simulink model "ADCS_model"  (R2019a)
settings: Solver=VariableStepAuto  StartTime=0.0  StopTime=10  RelTol=1e-3
undefined symbols (not defined in the file): A, As, c, Cd, f, G, J, JD_0, Jw, Ks, L, Ls, M, nut80, q
libraries: vrlib x5, dspmathops x1
(part 1 of 2)
settings Model: Creator=mario  LastModifiedBy=mario
settings DataIOCC: ReturnWorkspaceOutputs=off
settings DebuggingCC: ArithmeticOperatorsInVariantConditions=warning

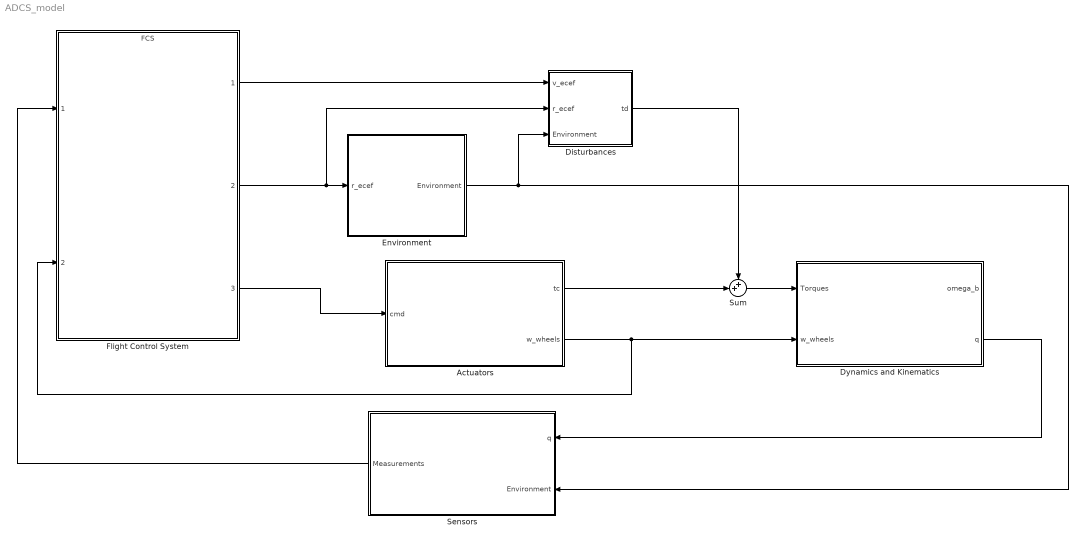
== system ADCS_model ==
  Actuators : Subsystem
  Disturbances : Subsystem
  "Dynamics and Kinematics " : Subsystem
  Environment : Subsystem
  Flight Control System : ModelReference  ModelNameDialog=FCS.slx  SimulationMode=Normal  ModelReferenceVersion=1.10
  Sensors : Subsystem
  Sum : Sum  Inputs=++|
  wires:
  "Dynamics and Kinematics "/2(q) -> Sensors/1(q)
  Sensors/1(Measurements) -> Flight Control System/1
  Disturbances/1(td) -> Sum/1
  Actuators/1(tc) -> Sum/2
  Environment/1(Environment) -> Sensors/2(Environment), Disturbances/3(Environment)
  Sum/1 -> "Dynamics and Kinematics "/1(Torques)
  Flight Control System/2 -> Environment/1(r_ecef), Disturbances/2("r_ecef ")
  Actuators/2(w_wheels) -> Flight Control System/2, "Dynamics and Kinematics "/2(w_wheels)
  Flight Control System/1 -> Disturbances/1(v_ecef)
  Flight Control System/3 -> Actuators/1(cmd)

== system ADCS_model/Actuators ==
  cmd : Inport
  Magnetorquers : Subsystem
  Reaction Wheels : Subsystem
  Sum : Sum
  tc : Outport  VectorParamsAs1DForOutWhenUnconnected=on
  w_wheels : Outport  Port=2  VectorParamsAs1DForOutWhenUnconnected=on
  wires:
  Reaction Wheels/1(t_wheels) -> Sum/1
  Reaction Wheels/2(w_wheels) -> w_wheels/1
  Magnetorquers/1(Out1) -> Sum/2
  Sum/1 -> tc/1
  cmd/1 -> Reaction Wheels/1(cmd_rpm)

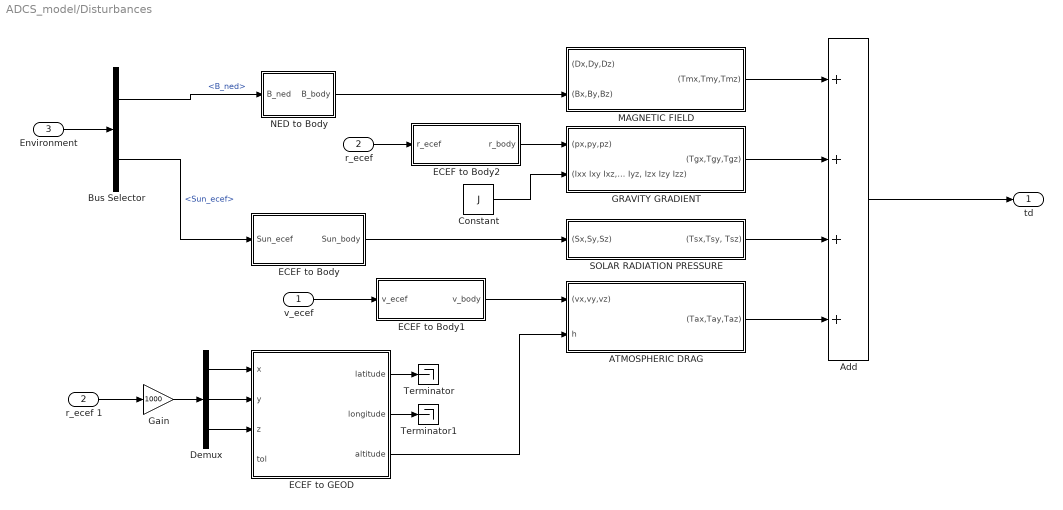
== system ADCS_model/Disturbances ==
  v_ecef : Inport
  "r_ecef " : Inport  Port=2
  Environment : Inport  Port=3
  ATMOSPHERIC DRAG : Subsystem
  Add : Sum  Inputs=4
  Bus Selector : BusSelector  OutputSignals=B_ned,Sun_ecef
  Constant : Constant  Value=J
  Demux : Demux  Outputs=3
  ECEF to Body : Subsystem
  ECEF to Body1 : Subsystem
  ECEF to Body2 : Subsystem
  ECEF to GEOD : MATLAB Function  TreatAsAtomicUnit=on
  GRAVITY GRADIENT : Subsystem
  Gain : Gain  Gain=1000
  "MAGNETIC FIELD " : Subsystem
  NED to Body : Subsystem
  SOLAR RADIATION PRESSURE : Subsystem
  Terminator : Terminator
  Terminator1 : Terminator
  r_ecef 1 : InportShadow  Port=2
  td : Outport
  wires:
  Add/1 -> td/1
  ECEF to GEOD/3(altitude) -> ATMOSPHERIC DRAG/2("h ")
  Constant/1 -> GRAVITY GRADIENT/2("(Ixx Ixy Ixz, Iyx Iyy Iyz, Izx Izy Izz)")
  ATMOSPHERIC DRAG/1((Tax,Tay,Taz)) -> Add/4
  GRAVITY GRADIENT/1((Tgx,Tgy,Tgz)) -> Add/2
  ? -> "MAGNETIC FIELD "/1((Dx,Dy,Dz))
  SOLAR RADIATION PRESSURE/1("(Tsx,Tsy, Tsz)") -> Add/3
  NED to Body/1(B_body) -> "MAGNETIC FIELD "/2((Bx,By,Bz))
  "MAGNETIC FIELD "/1((Tmx,Tmy,Tmz)) -> Add/1
  ECEF to Body/1(Sun_body) -> SOLAR RADIATION PRESSURE/1((Sx,Sy,Sz))
  ECEF to Body1/1(v_body) -> ATMOSPHERIC DRAG/1((vx,vy,vz))
  Environment/1 -> Bus Selector/1
  Bus Selector/1 -> NED to Body/1(B_ned)  "<B_ned>"
  Bus Selector/2 -> ECEF to Body/1(Sun_ecef)  "<Sun_ecef>"
  v_ecef/1 -> ECEF to Body1/1(v_ecef)
  "r_ecef "/1 -> ECEF to Body2/1(r_ecef)
  ECEF to Body2/1(r_body) -> GRAVITY GRADIENT/1((px,py,pz))
  r_ecef 1/1 -> Gain/1
  Demux/1 -> ECEF to GEOD/1(x)
  Demux/2 -> ECEF to GEOD/2(y)
  Demux/3 -> ECEF to GEOD/3(z)
  ECEF to GEOD/1(latitude) -> Terminator/1
  ECEF to GEOD/2(longitude) -> Terminator1/1
  Gain/1 -> Demux/1

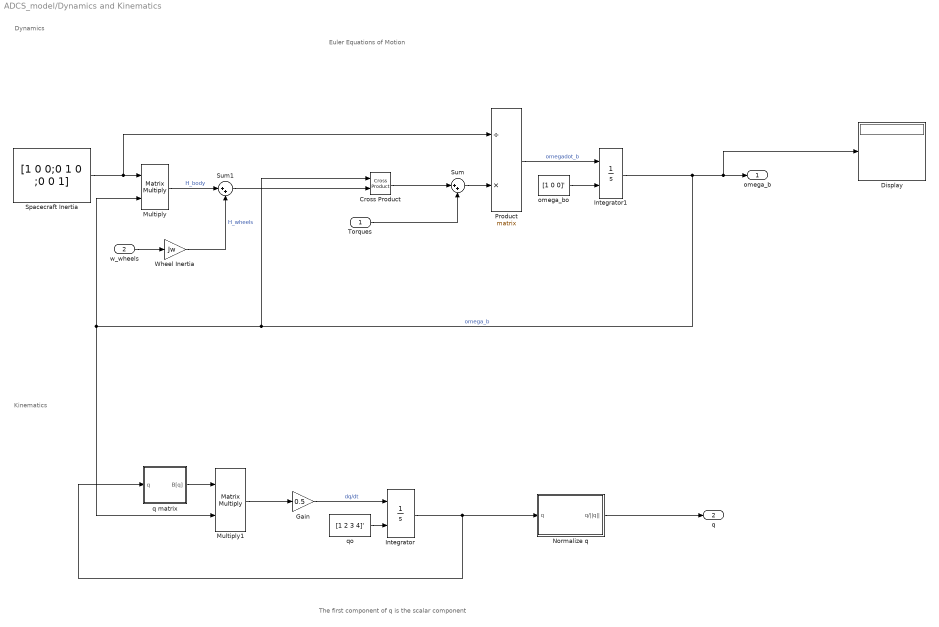
== system ADCS_model/Dynamics and Kinematics  ==
  note: Kinematics
  note: Dynamics
  note: Euler Equations of Motion
  note: The first component of q is the scalar component
  Torques : Inport
  w_wheels : Inport  Port=2
  Cross Product : vrlib/Utilities/Cross Product
      settings: SourceProductName=Simulink
  Display : Display
  Gain : Gain  Gain=0.5
  Integrator : Integrator  InitialConditionSource=external
  Integrator1 : Integrator  InitialConditionSource=external
  Multiply : Product  Multiplication=Matrix(*)
  Multiply1 : Product  Multiplication=Matrix(*)
  Normalize q : Subsystem
  Product : Product  Inputs=/*  Multiplication=Matrix(*)
  Spacecraft Inertia : Constant  Value=[1 0 0;0 1 0 ;0 0 1]
  Sum : Sum  Inputs=|++
  Sum1 : Sum  Inputs=|++
  Wheel Inertia : Gain  Gain=Jw
  omega_bo : Constant  Value=[1 0 0]'
  q matrix : Subsystem
  qo : Constant  Value=[1 2 3 4]'
  omega_b : Outport
  q : Outport  Port=2
  wires:
  Integrator1/1 -> Display/1, omega_b/1, Multiply1/2, Multiply/2, Cross Product/1  "omega_b"
  Spacecraft Inertia/1 -> Product/1, Multiply/1
  omega_bo/1 -> Integrator1/2
  Product/1 -> Integrator1/1  "omegadot_b"
  Multiply/1 -> Sum1/1  "H_body"
  Sum/1 -> Product/2
  Cross Product/1 -> Sum/1
  Sum1/1 -> Cross Product/2
  Wheel Inertia/1 -> Sum1/2  "H_wheels"
  w_wheels/1 -> Wheel Inertia/1
  Torques/1 -> Sum/2
  Multiply1/1 -> Gain/1
  Gain/1 -> Integrator/1  "dq/dt"
  Integrator/1 -> Normalize q/1(q), q matrix/1(q)
  q matrix/1(B[q]) -> Multiply1/1
  qo/1 -> Integrator/2
  Normalize q/1(q/||q||) -> q/1

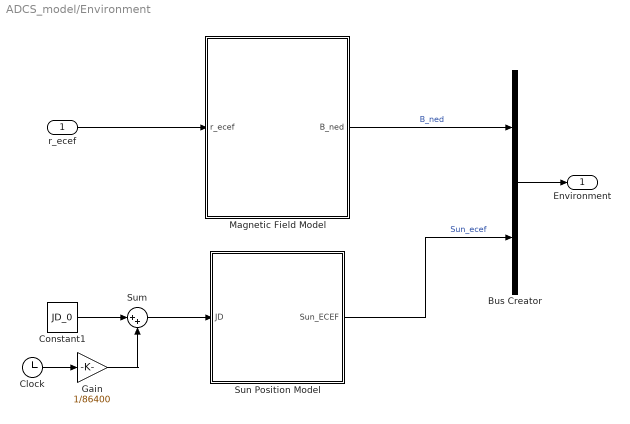
== system ADCS_model/Environment ==
  r_ecef : Inport
  Bus Creator : BusCreator  Inputs=2
  Clock : Clock
  Constant1 : Constant  Value=JD_0
  Gain : Gain  Gain=1/86400
  Magnetic Field Model : Subsystem
  Sum : Sum  Inputs=|++
  "Sun Position Model " : Subsystem
  Environment : Outport
  wires:
  Clock/1 -> Gain/1
  Constant1/1 -> Sum/1
  Gain/1 -> Sum/2
  Sum/1 -> "Sun Position Model "/1(JD)
  Magnetic Field Model/1(B_ned) -> Bus Creator/1  "B_ned"
  "Sun Position Model "/1(Sun_ECEF) -> Bus Creator/2  "Sun_ecef"
  Bus Creator/1 -> Environment/1
  r_ecef/1 -> Magnetic Field Model/1(r_ecef)

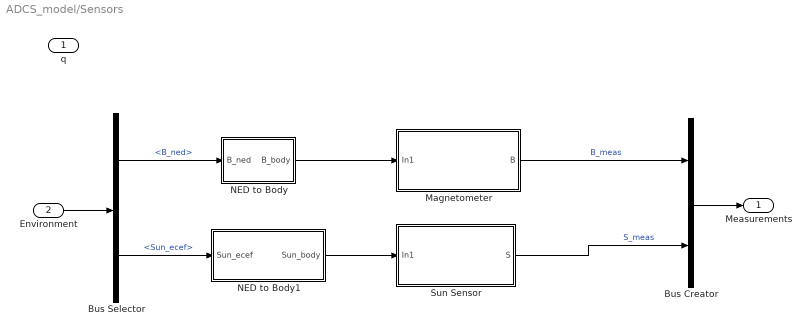
== system ADCS_model/Sensors ==
  q : Inport
  Environment : Inport  Port=2
  Bus Creator : BusCreator  Inputs=2
  Bus Selector : BusSelector  OutputSignals=B_ned,Sun_ecef
  Magnetometer : Subsystem
  NED to Body : Subsystem
  NED to Body1 : Subsystem
  Sun Sensor : Subsystem
  Measurements : Outport
  wires:
  Environment/1 -> Bus Selector/1
  Bus Selector/1 -> NED to Body/1(B_ned)  "<B_ned>"
  NED to Body/1(B_body) -> Magnetometer/1(In1)
  Magnetometer/1(B) -> Bus Creator/1  "B_meas"
  Bus Creator/1 -> Measurements/1
  Bus Selector/2 -> NED to Body1/1(Sun_ecef)  "<Sun_ecef>"
  NED to Body1/1(Sun_body) -> Sun Sensor/1(In1)
  Sun Sensor/1(S) -> Bus Creator/2  "S_meas"

== system ADCS_model/Actuators/Magnetorquers ==
  In1 : Inport
  Out1 : Outport
  wires:
  In1/1 -> Out1/1

== system ADCS_model/Actuators/Reaction Wheels ==
  cmd_rpm : Inport
  Demux : Demux  Outputs=3
  Mux : Mux  Inputs=3
  Mux1 : Mux  Inputs=3
  Reactionwheel_x : Subsystem
  Reactionwheel_y : Subsystem
  Reactionwheel_z : Subsystem
  t_wheels : Outport
  w_wheels : Outport  Port=2
  wires:
  Reactionwheel_y/1(t_wheels) -> Mux/2
  Reactionwheel_y/2(w_wheels) -> Mux1/2
  Demux/1 -> Reactionwheel_x/1(cmd_rpm)
  Reactionwheel_x/2(w_wheels) -> Mux1/1
  Demux/2 -> Reactionwheel_y/1(cmd_rpm)
  Demux/3 -> Reactionwheel_z/1(cmd_rpm)
  Reactionwheel_z/2(w_wheels) -> Mux1/3
  Reactionwheel_x/1(t_wheels) -> Mux/1
  Reactionwheel_z/1(t_wheels) -> Mux/3
  Mux1/1 -> w_wheels/1
  Mux/1 -> t_wheels/1
  cmd_rpm/1 -> Demux/1

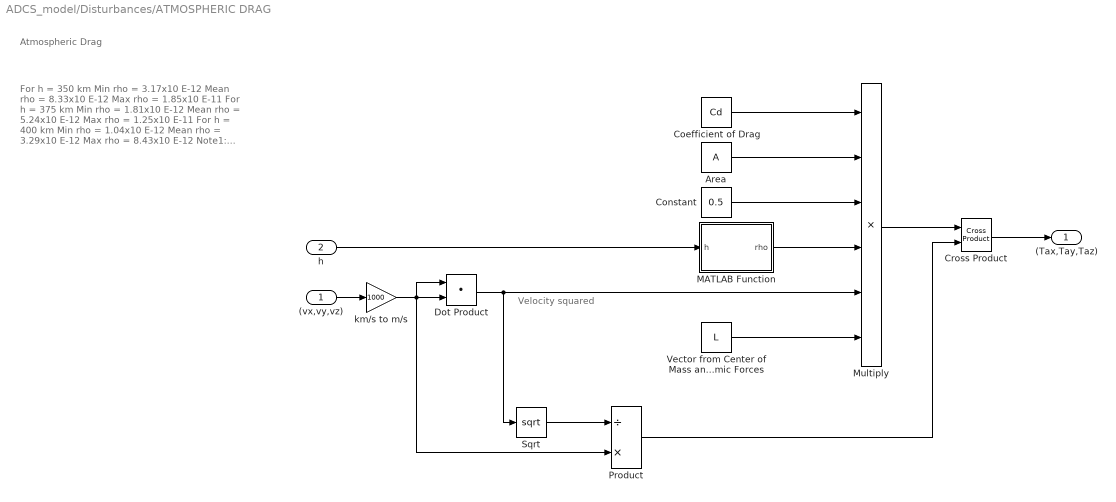
== system ADCS_model/Disturbances/ATMOSPHERIC DRAG ==
  note: Velocity squared
  note: For h = 350 km
      |
      | Min rho = 3.17x10 E-12
      | Mean rho = 8.33x10 E-12
      | Max rho = 1.85x10 E-11
      |
      | For h = 375 km
      |
      | Min rho = 1.81x10 E-12
      | Mean rho = 5.24x10 E-12
      | Max rho = 1.25x10 E-11
      |
      | For h = 400 km
      |
      | Min rho = 1.04x10 E-12
      | Mean rho = 3.29x10 E-12
      | Max rho = 8.43x10 E-12
      |
      | Note1: Mean Rho has an accuracy of 10%
      | Note2: Rho (kg/m^3)
      | Note3 : Rho depends on solar pressure and the solar cycle
      | Source : New SMAD p.1031
  note: Atmospheric Drag
  (vx,vy,vz) : Inport
  "h " : Inport  Port=2
  Area : Constant  Value=A
  Coefficient of Drag : Constant  Value=Cd
  Constant : Constant  Value=0.5
  Cross Product : vrlib/Utilities/Cross Product
      settings: SourceProductBaseCode=VR
  Dot Product : DotProduct  InputSameDT=on  OutDataTypeStr=Inherit: Inherit via internal rule
  MATLAB Function : MATLAB Function  TreatAsAtomicUnit=on
  Multiply : Product  Inputs=6
  Product : Product  Inputs=/*
  Sqrt : Sqrt  SaturateOnIntegerOverflow=on
  "Vector from Center of Mass and Center of Aerodynamic Forces " : Constant  Value=L
  km/s to m/s : Gain  Gain=1000
  (Tax,Tay,Taz) : Outport
  wires:
  Constant/1 -> Multiply/3
  Multiply/1 -> Cross Product/1
  (vx,vy,vz)/1 -> km/s to m/s/1
  "h "/1 -> MATLAB Function/1(h)
  Sqrt/1 -> Product/1
  Product/1 -> Cross Product/2
  Dot Product/1 -> Sqrt/1, Multiply/5
  Area/1 -> Multiply/2
  Coefficient of Drag/1 -> Multiply/1
  MATLAB Function/1(rho) -> Multiply/4
  "Vector from Center of Mass and Center of Aerodynamic Forces "/1 -> Multiply/6
  Cross Product/1 -> (Tax,Tay,Taz)/1
  km/s to m/s/1 -> Dot Product/1, Product/2, Dot Product/2

== system ADCS_model/Disturbances/ECEF to Body ==
  Sun_ecef : Inport
  Sun_body : Outport
  wires:
  Sun_ecef/1 -> Sun_body/1

== system ADCS_model/Disturbances/ECEF to Body1 ==
  v_ecef : Inport
  v_body : Outport
  wires:
  v_ecef/1 -> v_body/1

== system ADCS_model/Disturbances/ECEF to Body2 ==
  r_ecef : Inport
  r_body : Outport
  wires:
  r_ecef/1 -> r_body/1

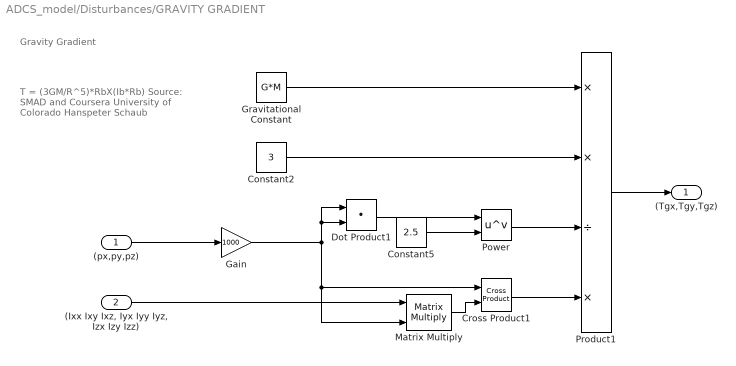
== system ADCS_model/Disturbances/GRAVITY GRADIENT ==
  note: T = (3GM/R^5)*RbX(Ib*Rb)
      |
      | Source: SMAD and Coursera
      | University of Colorado Hanspeter
      | Schaub
  note: Gravity Gradient
  (px,py,pz) : Inport
  "(Ixx Ixy Ixz, Iyx Iyy Iyz, Izx Izy Izz)" : Inport  Port=2
  Constant2 : Constant  Value=3
  Constant5 : Constant  Value=2.5
  Cross Product1 : vrlib/Utilities/Cross Product
      settings: SourceProductBaseCode=VR
  Dot Product1 : DotProduct  InputSameDT=on  OutDataTypeStr=Inherit: Inherit via internal rule
  Gain : Gain  Gain=1000
  Gravitational Constant : Constant  Value=G*M
  Matrix Multiply : Product  Multiplication=Matrix(*)
  Power : Math  Operator=pow  SaturateOnIntegerOverflow=on
  Product1 : Product  Inputs=**/*
  (Tgx,Tgy,Tgz) : Outport
  wires:
  (px,py,pz)/1 -> Gain/1
  Dot Product1/1 -> Power/1
  Constant5/1 -> Power/2
  Cross Product1/1 -> Product1/4
  Constant2/1 -> Product1/2
  "(Ixx Ixy Ixz, Iyx Iyy Iyz, Izx Izy Izz)"/1 -> Matrix Multiply/1
  Matrix Multiply/1 -> Cross Product1/2
  Gravitational Constant/1 -> Product1/1
  Power/1 -> Product1/3
  Product1/1 -> (Tgx,Tgy,Tgz)/1
  Gain/1 -> Matrix Multiply/2, Cross Product1/1, Dot Product1/1, Dot Product1/2

== system ADCS_model/Disturbances/MAGNETIC FIELD  ==
  note: Magnetic Field
  (Dx,Dy,Dz) : Inport
  (Bx,By,Bz) : Inport  Port=2
  Cross Product : vrlib/Utilities/Cross Product
      settings: SourceProductBaseCode=VR
  nT to T : Gain  Gain=1e-9
  (Tmx,Tmy,Tmz) : Outport
  wires:
  Cross Product/1 -> (Tmx,Tmy,Tmz)/1
  (Bx,By,Bz)/1 -> nT to T/1
  (Dx,Dy,Dz)/1 -> Cross Product/1
  nT to T/1 -> Cross Product/2

== system ADCS_model/Disturbances/NED to Body ==
  B_ned : Inport
  B_body : Outport
  wires:
  B_ned/1 -> B_body/1

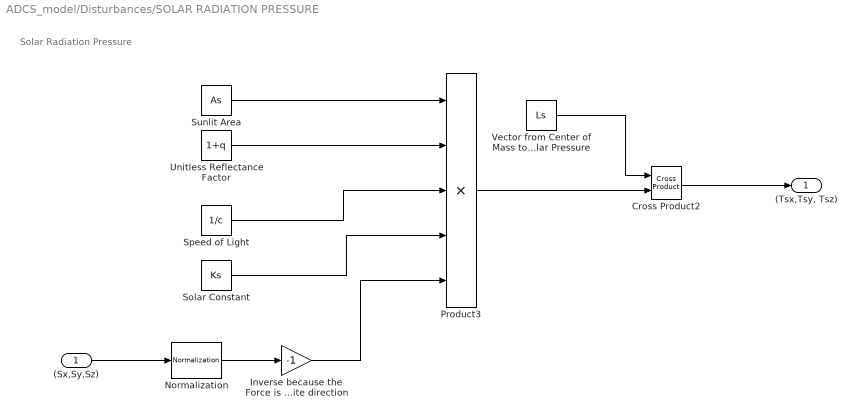
== system ADCS_model/Disturbances/SOLAR RADIATION PRESSURE ==
  note: Solar Radiation
      | Pressure
  (Sx,Sy,Sz) : Inport
  Cross Product2 : vrlib/Utilities/Cross Product
      settings: SourceProductBaseCode=VR
  Inverse because the Force is in the opposite direction : Gain  Gain=-1
  Normalization : dspmathops/Normalization  NormType=2-norm  Bias=1e-10  NormOver=Each column  Dimension=1  roundingMode=Floor  overflowMode=off  accumDataTypeStr=Inherit: Same as product output  accumLastDataTypeStr=Inherit: Same as product output  outputDataTypeStr=Inherit: Same as product output  outputMin=[]  outputMax=[]  outputLastDataTypeStr=Inherit: Same as product output
      settings: SourceProductName=DSP System Toolbox
  Product3 : Product  Inputs=5
  Solar Constant : Constant  Value=Ks
  Speed of Light : Constant  Value=1/c
  Sunlit Area : Constant  Value=As
  Unitless Reflectance Factor : Constant  Value=1+q
  Vector from Center of Mass to Center of Solar Pressure : Constant  Value=Ls
  "(Tsx,Tsy, Tsz)" : Outport
  wires:
  Cross Product2/1 -> "(Tsx,Tsy, Tsz)"/1
  Sunlit Area/1 -> Product3/1
  Vector from Center of Mass to Center of Solar Pressure/1 -> Cross Product2/1
  (Sx,Sy,Sz)/1 -> Normalization/1
  Solar Constant/1 -> Product3/4
  Product3/1 -> Cross Product2/2
  Inverse because the Force is in the opposite direction/1 -> Product3/5
  Speed of Light/1 -> Product3/3
  Unitless Reflectance Factor/1 -> Product3/2
  Normalization/1 -> Inverse because the Force is in the opposite direction/1

== system ADCS_model/Dynamics and Kinematics /Normalize q ==
  q : Inport
  Divide : Product  Inputs=*/
  Dot Product : DotProduct  InputSameDT=on  OutDataTypeStr=Inherit: Inherit via internal rule
  Sqrt : Sqrt  SaturateOnIntegerOverflow=on
  q/||q|| : Outport
  wires:
  q/1 -> Divide/1, Dot Product/2, Dot Product/1
  Sqrt/1 -> Divide/2
  Dot Product/1 -> Sqrt/1
  Divide/1 -> q/||q||/1

== system ADCS_model/Dynamics and Kinematics /q matrix ==
  q : Inport
  Gain : Gain  Gain=[1 0 0 0;0 -1 0 0;0 0 -1 0;0 0 0 1]  Multiplication=Matrix(K*u)
  Gain1 : Gain  Gain=[1 0 0 0;0 1 0 0;0 0 -1 0;0 0 0 -1]  Multiplication=Matrix(K*u)
  Gain4 : Gain  Gain=[1 0 0 0;0 -1 0 0;0 0 1 0;0 0 0 -1]  Multiplication=Matrix(K*u)
  Matrix Concatenate : Concatenate  NumInputs=3  Mode=Multidimensional array  ConcatenateDimension=2
  Selector : Selector  InputPortWidth=4  IndexOptions=Index vector (dialog)  Indices=[2 1 4 3]  OutputSizes=1
  Selector2 : Selector  InputPortWidth=4  IndexOptions=Index vector (dialog)  Indices=[3 4 1 2]  OutputSizes=1
  Selector4 : Selector  InputPortWidth=4  IndexOptions=Index vector (dialog)  Indices=[4 3 2 1]  OutputSizes=1
  B[q] : Outport
  wires:
  Gain4/1 -> Selector4/1
  Selector2/1 -> Matrix Concatenate/2
  Matrix Concatenate/1 -> B[q]/1
  Selector4/1 -> Matrix Concatenate/3
  q/1 -> Gain4/1, Gain/1, Gain1/1
  Selector/1 -> Matrix Concatenate/1
  Gain1/1 -> Selector2/1
  Gain/1 -> Selector/1

== system ADCS_model/Environment/Magnetic Field Model ==
  r_ecef : Inport
  Demux : Demux  Outputs=3
  ECEF to GEOD : MATLAB Function  TreatAsAtomicUnit=on
  IGRF 13th Gen. : MATLAB Function  TreatAsAtomicUnit=on
  Mux : Mux  Inputs=3
  km to m : Gain  Gain=1000
  B_ned : Outport  VectorParamsAs1DForOutWhenUnconnected=on
  wires:
  ECEF to GEOD/3(altitude) -> IGRF 13th Gen./3(altitude)
  IGRF 13th Gen./2(Be) -> Mux/2
  IGRF 13th Gen./3(Bd) -> Mux/3
  ECEF to GEOD/2(longitude) -> IGRF 13th Gen./2(longitude)
  Demux/2 -> ECEF to GEOD/2(y)
  IGRF 13th Gen./1(Bn) -> Mux/1
  ECEF to GEOD/1(latitude) -> IGRF 13th Gen./1(latitude)
  Demux/3 -> ECEF to GEOD/3(z)
  Demux/1 -> ECEF to GEOD/1(x)
  r_ecef/1 -> km to m/1
  Mux/1 -> B_ned/1
  km to m/1 -> Demux/1

== system ADCS_model/Environment/Sun Position Model  ==
  JD : Inport
  MOD to ECEF : Subsystem
  Sun Position Vector : MATLAB Function  TreatAsAtomicUnit=on
  Sun_ECEF : Outport
  wires:
  Sun Position Vector/1(rsun) -> MOD to ECEF/1(Sun_MOD)
  JD/1 -> MOD to ECEF/2(JD), Sun Position Vector/1(jd)
  MOD to ECEF/1(Sun_ECEF) -> Sun_ECEF/1

== system ADCS_model/Sensors/Magnetometer ==
  In1 : Inport
  B : Outport
  wires:
  In1/1 -> B/1

== system ADCS_model/Sensors/NED to Body ==
  B_ned : Inport
  B_body : Outport
  wires:
  B_ned/1 -> B_body/1

== system ADCS_model/Sensors/NED to Body1 ==
  Sun_ecef : Inport
  Sun_body : Outport
  wires:
  Sun_ecef/1 -> Sun_body/1

== system ADCS_model/Sensors/Sun Sensor ==
  In1 : Inport
  S : Outport
  wires:
  In1/1 -> S/1

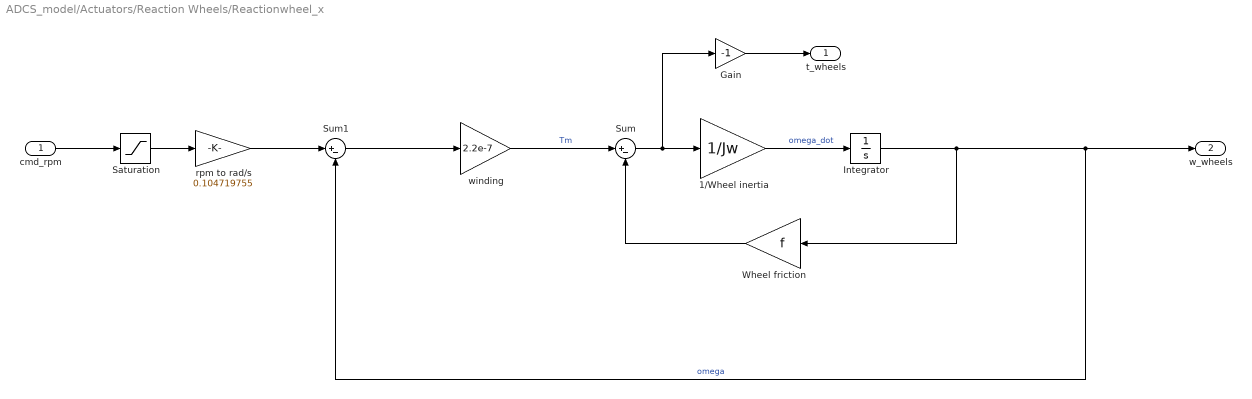
== system ADCS_model/Actuators/Reaction Wheels/Reactionwheel_x ==
  cmd_rpm : Inport
  1/Wheel inertia : Gain  Gain=1/Jw
  Gain : Gain  Gain=-1
  Integrator : Integrator
  Saturation : Saturate  UpperLimit=8000  LowerLimit=-8000
  Sum : Sum  Inputs=|+-
  Sum1 : Sum  Inputs=|+-
  Wheel friction : Gain  Gain=f
  rpm to rad/s : Gain  Gain=0.104719755
  winding : Gain  Gain=2.2e-7
  t_wheels : Outport
  w_wheels : Outport  Port=2
  wires:
  cmd_rpm/1 -> Saturation/1
  Integrator/1 -> w_wheels/1, Sum1/2, Wheel friction/1  "omega"
  Wheel friction/1 -> Sum/2
  Sum1/1 -> winding/1
  1/Wheel inertia/1 -> Integrator/1  "omega_dot"
  winding/1 -> Sum/1  "Tm"
  Sum/1 -> Gain/1, 1/Wheel inertia/1
  rpm to rad/s/1 -> Sum1/1
  Saturation/1 -> rpm to rad/s/1
  Gain/1 -> t_wheels/1

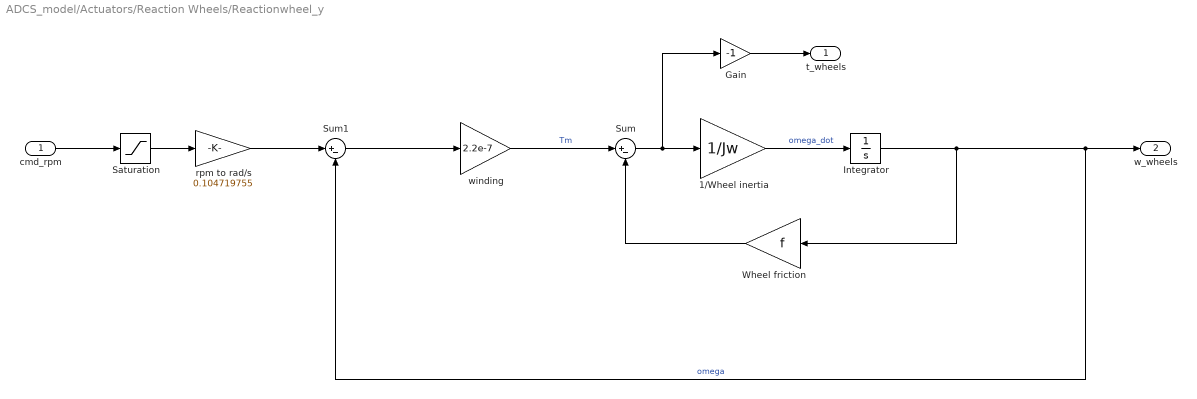
== system ADCS_model/Actuators/Reaction Wheels/Reactionwheel_y ==
  cmd_rpm : Inport
  1/Wheel inertia : Gain  Gain=1/Jw
  Gain : Gain  Gain=-1
  Integrator : Integrator
  Saturation : Saturate  UpperLimit=8000  LowerLimit=-8000
  Sum : Sum  Inputs=|+-
  Sum1 : Sum  Inputs=|+-
  Wheel friction : Gain  Gain=f
  rpm to rad/s : Gain  Gain=0.104719755
  winding : Gain  Gain=2.2e-7
  t_wheels : Outport
  w_wheels : Outport  Port=2
  wires:
  Saturation/1 -> rpm to rad/s/1
  rpm to rad/s/1 -> Sum1/1
  Sum/1 -> 1/Wheel inertia/1, Gain/1
  winding/1 -> Sum/1  "Tm"
  1/Wheel inertia/1 -> Integrator/1  "omega_dot"
  Sum1/1 -> winding/1
  Wheel friction/1 -> Sum/2
  Integrator/1 -> Wheel friction/1, w_wheels/1, Sum1/2  "omega"
  cmd_rpm/1 -> Saturation/1
  Gain/1 -> t_wheels/1

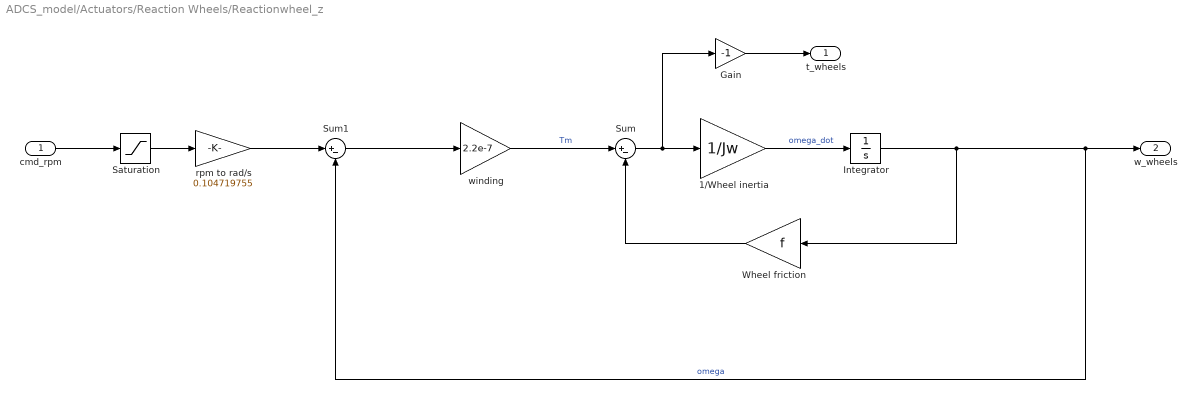
== system ADCS_model/Actuators/Reaction Wheels/Reactionwheel_z ==
  cmd_rpm : Inport
  1/Wheel inertia : Gain  Gain=1/Jw
  Gain : Gain  Gain=-1
  Integrator : Integrator
  Saturation : Saturate  UpperLimit=8000  LowerLimit=-8000
  Sum : Sum  Inputs=|+-
  Sum1 : Sum  Inputs=|+-
  Wheel friction : Gain  Gain=f
  rpm to rad/s : Gain  Gain=0.104719755
  winding : Gain  Gain=2.2e-7
  t_wheels : Outport
  w_wheels : Outport  Port=2
  wires:
  cmd_rpm/1 -> Saturation/1
  Integrator/1 -> Sum1/2, w_wheels/1, Wheel friction/1  "omega"
  Wheel friction/1 -> Sum/2
  Sum1/1 -> winding/1
  1/Wheel inertia/1 -> Integrator/1  "omega_dot"
  winding/1 -> Sum/1  "Tm"
  Sum/1 -> Gain/1, 1/Wheel inertia/1
  rpm to rad/s/1 -> Sum1/1
  Saturation/1 -> rpm to rad/s/1
  Gain/1 -> t_wheels/1

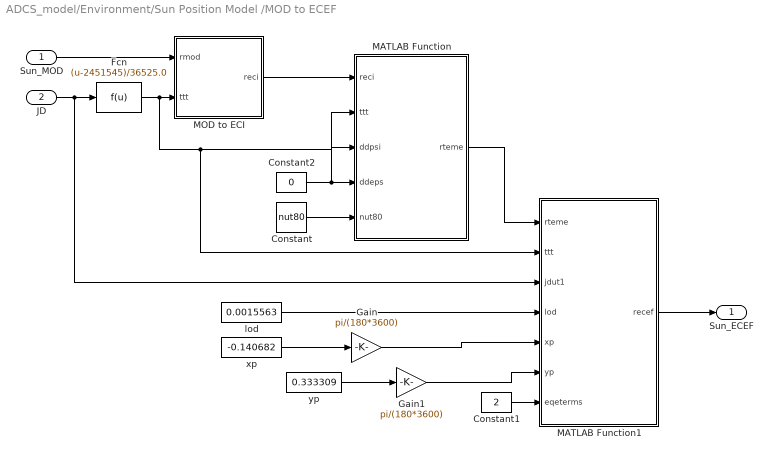
== system ADCS_model/Environment/Sun Position Model /MOD to ECEF ==
  Sun_MOD : Inport
  JD : Inport  Port=2
  Constant : Constant  Value=nut80
  Constant1 : Constant  Value=2
  Constant2 : Constant  Value=0
  Fcn : Fcn  Expr=(u-2451545)/36525.0
  Gain : Gain  Gain=pi/(180*3600)
  Gain1 : Gain  Gain=pi/(180*3600)
  MATLAB Function : MATLAB Function  TreatAsAtomicUnit=on
  MATLAB Function1 : MATLAB Function  TreatAsAtomicUnit=on
  MOD to ECI : MATLAB Function  TreatAsAtomicUnit=on
  lod : Constant  Value=0.0015563
  xp : Constant  Value=-0.140682
  yp : Constant  Value=0.333309
  Sun_ECEF : Outport
  wires:
  Sun_MOD/1 -> MOD to ECI/1(rmod)
  Fcn/1 -> MATLAB Function1/2(ttt), MATLAB Function/2(ttt), MOD to ECI/2(ttt)
  JD/1 -> MATLAB Function1/3(jdut1), Fcn/1
  MOD to ECI/1(reci) -> MATLAB Function/1(reci)
  Constant2/1 -> MATLAB Function/4(ddeps), MATLAB Function/3(ddpsi)
  MATLAB Function1/1(recef) -> Sun_ECEF/1
  MATLAB Function/1(rteme) -> MATLAB Function1/1(rteme)
  Constant/1 -> MATLAB Function/5(nut80)
  Constant1/1 -> MATLAB Function1/7(eqeterms)
  lod/1 -> MATLAB Function1/4(lod)
  Gain/1 -> MATLAB Function1/5(xp)
  yp/1 -> Gain1/1
  xp/1 -> Gain/1
  Gain1/1 -> MATLAB Function1/6(yp)

== matlab function ADCS_model/Environment/Sun Position Model /MOD to ECEF/MOD to ECI ==
  data: rmod input; reci output; ttt input
% ----------------------------------------------------------------------------
%
%                           function mod2eci
%
%  this function transforms a vector from the mean equator mean equinox of
%    date (mod) to the mean equator mean equinox (j2000) frame.
%
%  author        : david vallado                  719-573-2600   25 jun 2002
%
%  revisions
%    vallado     - consolidate with iau 2000                     14 feb 2005
%
%  inputs          description                    range / units
%    rmod        - position vector of date
%                    mean equator, mean equinox   km
%    vmod        - velocity vector of date
%                    mean equator, mean equinox   km/s
%    amod        - acceleration vector of date
%                    mean equator, mean equinox   km/s2
%    ttt         - julian centuries of tt         centuries
%
%  outputs       :
%    reci        - position vector eci            km
%    veci        - velocity vector eci            km/s
%    aeci        - acceleration vector eci        km/s2
%
%  locals        :
%    none.
%
%  coupling      :
%   precess      - rotation for precession        mod - eci
%
%  references    :
%    vallado       2001, 219-220, eq 3-68
%
% [reci,veci,aeci] = mod2eci  ( rmod,vmod,amod,ttt );
% ----------------------------------------------------------------------------

function reci  = mod2eci  ( rmod,ttt )
        
        
        [prec,psia,wa,ea,xa] = precess1 ( ttt);

        reci = prec*rmod;
        
        
        
        
        % ----------------------------------------------------------------------------
%
%                           function precess
%
%  this function calulates the transformation matrix that accounts for the effects
%    of precession. both the 1980 and 2000 theories are handled. note that the 
%    required parameters differ a little. 
%
%  author        : david vallado                  719-573-2600   25 jun 2002
%
%  revisions
%    vallado     - consolidate with iau 2000                     14 feb 2005
%
%  inputs          description                    range / units
%    ttt         - julian centuries of tt
%    opt         - method option                  '01', '02', '96', '80'
%
%  outputs       :
%    prec        - transformation matrix for mod - j2000 (80 only)
%    psia        - cannonical precession angle    rad    (00 only)
%    wa          - cannonical precession angle    rad    (00 only)
%    ea          - cannonical precession angle    rad    (00 only)
%    xa          - cannonical precession angle    rad    (00 only)
%
%  locals        :
%    ttt2        - ttt squared
%    ttt3        - ttt cubed
%    zeta        - precession angle               rad
%    z           - precession angle               rad
%    theta       - precession angle               rad
%    oblo        - obliquity value at j2000 epoch "%
%
%  coupling      :
%    none        -
%
%  references    :
%    vallado       2004, 214-216, 219-221
%
% [prec,psia,wa,ea,xa] = precess ( ttt, opt );
% ----------------------------------------------------------------------------

function [prec,psia,wa,ea,xa] = precess1 ( ttt );

       % sethelp;
        
        % " to rad
        convrt = pi / (180.0*3600.0);
        ttt2= ttt * ttt;
        ttt3= ttt2 * ttt;

        % ------------------- fk4 b1950 precession angles --------------------
%         if (opt == '50')
% 
%             % ---- Seidelmann pg 107             
%             % for these calls, ttt will come in with the current jd
% %            t1= 0.0; %(ttt - 2433282.42345905)/365242.198782;  % set start as B1850, 0.0 to simplify
% %            t2= (ttt - 2396758.203)/365242.198782;  % uses B1850
% %            ttt = t2 - t1;
% %            ttt2 = ttt * ttt;
% %            ttt3 = ttt * ttt2;
% %            fprintf(1,'50prec %15.9f  \n',ttt);
%             % exp supp 61 pg 38
% %            psia = 50.3708 + 0.0050 * ttt;
% %            wa = 0.0;
% %            ea = 0.0;
% %            xa = 0.1247 - 0.0188 * ttt;
% %            zeta =  (23035.545 + 139.720*t1 + 0.060 *t1*t1)*ttt + (30.240-0.270*t1)*ttt2 + 17.995*ttt3; % "
% %            theta=  (20051.12 - 85.29*t1 - 0.37 *t1*t1)*ttt + (-42.65-0.37*t1)*ttt2 - 41.80*ttt3;
% %            z    =  (23035.545 + 139.720*t1 + 0.060 *t1*t1)*ttt + (109.480+0.390*t1)*ttt2 + 18.325*ttt3;
% 
%             % ---- Newcomb Exp Supp 61 approach, but see GTDS pg 3-17
%             % Exp Supp 61 says use 1900? but gtds says use 1950. 
%             % for these calls, ttt will come in with the current jd
%             t1= 0.0; %(ttt - 2415020.31352)/36524.2198782;  % set start as B1900, 0.0 to simplify
% %            t2= (ttt - 2415020.31352)/36525;  % uses B1900   
%             t2= (ttt - 2433282.42345905)/36525;  % uses B1950  
% %            ttt = t2 - t1;
% %            ttt2 = ttt * ttt;
% %            ttt3 = ttt * ttt2;
%             % exp supp 61 pg 38
%             psia = 50.3708 + 0.0050 * ttt;
%             wa = 0.0; % not sure which one is which...
%             ea = 84428.26 -   46.845*ttt - 0.00059*ttt2 + 0.00181*ttt3;
%             xa = 0.1247 - 0.0188 * ttt;
%            fprintf(1,'50prec %15.9f  \n',ttt);
%            % seems like Exp supp 61 is ok with 1900 as epoch, and Seidlemann is ok with listed measr,  
% %            zeta =  (2304.25 + 1.396*t1)*ttt + 0.302*ttt2 + 0.018*ttt3; % "
% %            theta=  (2004.682 - 0.853*t1)*ttt -0.426*ttt2 - 0.042*ttt3;
% %            z    =  (2304.25 + 1.396*t1)*ttt + 1.093*ttt2 + 0.018*ttt3;
%             % GTDS pg 3-17 using days from 1950 - avoids long rpecession
%             % constants...
%             zeta =  2304.9969*ttt + 0.302*ttt2 + 0.01808*ttt3; % "
%             theta=  2004.2980*ttt -0.425936*ttt2 - 0.0416*ttt3;
%             z    =  2304.9969*ttt + 1.092999*ttt2 + 0.0192*ttt3;
%             
% 
%             % tp-008 36-45
%             % ttt is tropical centruies from 1950 36524.22 days
%             prec = zeros(3,3);
%             prec(1,1) =  1.0 - 2.9696e-4 * ttt2 - 1.3e-7 * ttt3;
%             prec(1,2) =  2.234941e-2 * ttt + 6.76e-6 * ttt2 - 2.21e-6 * ttt3;
%             prec(1,3) =  9.7169e-3 * ttt - 2.07e-6 * ttt2 - 9.6e-7 * ttt3;
%             prec(2,1) =  -prec(1,2);
%             prec(2,2) =  1.0 - 2.4975e-4 * ttt2 - 1.5e-7 * ttt3;
%             prec(2,3) =  - 1.0858e-4 * ttt2;
%             prec(3,1) =  -prec(1,3);
%             prec(3,2) =  prec(2,3);
%             prec(3,3) =  1.0 - 4.721e-5 * ttt2;
%  
%             
%            % pass these back out for testing
%            psia = zeta;
%            wa = theta;
%            ea = z;
%         % ------------------- iau 76 precession angles --------------------
%         else
%           if (opt == '80')
%     fprintf(1,'80prec %15.9f  \n',ttt);
            psia =             5038.7784*ttt - 1.07259*ttt2 - 0.001147*ttt3; % "
            wa   = 84381.448                 + 0.05127*ttt2 - 0.007726*ttt3;
            ea   = 84381.448 -   46.8150*ttt - 0.00059*ttt2 + 0.001813*ttt3;
            xa   =               10.5526*ttt - 2.38064*ttt2 - 0.001125*ttt3;
            zeta =             2306.2181*ttt + 0.30188*ttt2 + 0.017998*ttt3; % "
            theta=             2004.3109*ttt - 0.42665*ttt2 - 0.041833*ttt3;
            z    =             2306.2181*ttt + 1.09468*ttt2 + 0.018203*ttt3;
          % ------------------ iau 03 precession angles -------------------
%           else
%             oblo =  84381.406; % "
%             psia =  (((( -0.0000000951 * ttt + 0.000132851 ) * ttt - 0.00114045 ) * ttt - 1.0790069 ) * ttt + 5038.481507 ) * ttt; % "
%             wa   =  ((((  0.0000003337 * ttt - 0.000000467 ) * ttt - 0.00772503 ) * ttt + 0.0512623 ) * ttt -    0.025754 ) * ttt + oblo;
%             ea   =  (((( -0.0000000434 * ttt - 0.000000576 ) * ttt + 0.00200340 ) * ttt - 0.0001831 ) * ttt -   46.836769 ) * ttt + oblo;
%             xa   =  (((( - 0.0000000560 * ttt + 0.000170663 ) * ttt - 0.00121197 ) * ttt - 2.3814292 ) * ttt +   10.556403 ) * ttt;
% 
%             zeta =  (((( - 0.0000003173 * ttt - 0.000005971 ) * ttt + 0.01801828 ) * ttt + 0.2988499 ) * ttt + 2306.083227 ) * ttt + 2.650545; % "
%             theta=  (((( - 0.0000001274 * ttt - 0.000007089 ) * ttt - 0.04182264 ) * ttt - 0.4294934 ) * ttt + 2004.191903 ) * ttt;
%             z    =  ((((   0.0000002904 * ttt - 0.000028596 ) * ttt + 0.01826837 ) * ttt + 1.0927348 ) * ttt + 2306.077181 ) * ttt - 2.650545;
%           end;
%         end;
        
        % convert units to rad
        psia = psia  * convrt; % rad
        wa   = wa    * convrt;
        ea   = ea    * convrt;
        xa   = xa    * convrt;
        zeta = zeta  * convrt; 
        theta= theta * convrt;
        z    = z     * convrt;
%iauhelp='y';         
%fprintf(1,'pr %11.7f  %11.7f  %11.7fdeg \n',zeta*180/pi,theta*180/pi,z*180/pi );
%         if (iauhelp == 'y')
%             fprintf(1,'pr %11.7f  %11.7f  %11.7f %11.7fdeg \n',psia*180/pi,wa*180/pi,ea*180/pi,xa*180/pi );
%             fprintf(1,'pr %11.7f  %11.7f  %11.7fdeg \n',zeta*180/pi,theta*180/pi,z*180/pi );
%         end;
% 
%         if (strcmp(opt,'80')==1) % || (strcmp(opt,'50') == 1)
            coszeta  = cos(zeta);
            sinzeta  = sin(zeta);
            costheta = cos(theta);
            sintheta = sin(theta);
            cosz     = cos(z);
            sinz     = sin(z);

            % ----------------- form matrix  mod to j2000 -----------------
            prec = zeros(3,3);
            prec(1,1) =  coszeta * costheta * cosz - sinzeta * sinz;
            prec(1,2) =  coszeta * costheta * sinz + sinzeta * cosz;
            prec(1,3) =  coszeta * sintheta;
            prec(2,1) = -sinzeta * costheta * cosz - coszeta * sinz;
            prec(2,2) = -sinzeta * costheta * sinz + coszeta * cosz;
            prec(2,3) = -sinzeta * sintheta;
            prec(3,1) = -sintheta * cosz;
            prec(3,2) = -sintheta * sinz;
            prec(3,3) =  costheta;

== matlab function ADCS_model/Environment/Magnetic Field Model/IGRF 13th Gen. ==
  data: latitude input; Bn output; longitude input; altitude input; Be output; Bd output
function [Bn, Be, Bd] = igrf(latitude, longitude, altitude)

%REMOVED COORD AS EVERYTHING IS ALREADY IN GEOCENTRIC. KEEPING TIME FOR NOW

% IGRF Earth's magnetic field from IGRF model.
% 
% Usage: [BX, BY, BZ] = IGRF(TIME, LATITUDE, LONGITUDE, ALTITUDE, COORD)
%     or [BX, BY, BZ] = IGRF(COEFS, LATITUDE, LONGITUDE, ALTITUDE, COORD)
%     or B = IGRF(TIME, LATITUDE, LONGITUDE, ALTITUDE, COORD)
%     or B = IGRF(COEFS, LATITUDE, LONGITUDE, ALTITUDE, COORD)
% 
% Calculates the components of the Earth's magnetic field using the
% International Geomagnetic Reference Field (IGRF) model. The inputs for
% the position can be scalars or vectors (in the latter case each should
% have the same number of elements or be a scalar), but TIME must be a
% scalar.
% 
% When all the coordinate inputs are scalars, the function can be run more
% efficiently by providing the proper IGRF coefficient vector for a given
% time rather than the time itself. This mode is useful when making
% multiple calls to the function while keeping the time the same (meaning
% the coefficients will be the same for each run) as loading the
% coefficients can be the most time-consuming part of the function. The
% coefficient vector can be easily loaded using the function LOADIGRFCOEFS.
% This mode is assumed when all the coordinate inputs are scalars and the
% first input is a vector. In this case, the coefficient vector should be
% formatted as (LOADIGRFCOEFS provides this):
% 
%   [g(n=1,m=0) g(n=1,m=1) h(n=1,m=1) g(n=2,m=0) g(n=2,m=1) h(n=2,m=1) ...]
% 
% Regardless of the size of the inputs, the outputs will be column vectors.
% If only one output is requested, B = [BX(:), BY(:), BZ(:)] is output.
% Note that the other parameters the IGRF gives can be computed from BX,
% BY, and BZ as:
% 
%   Horizonal intensity: hypot(BX, BY) (i.e., sqrt(BX.^2 + BY.^2) )
%   Total intensity: hypot(BX, hypot(BY, BZ))
%   Declination: atan2(BY, BX)
%   Inclination: atan(BZ./hypot(BX, BY))
% 
% This function relies on having the file igrfcoefs.mat in the MATLAB
% path to function properly when a time is input. If this file cannot be
% found, this function will try to create it by calling GETIGRFCOEFS.
% 
% The IGRF is a spherical harmonic expansion of the Earth's internal
% magnetic field. Currently, the IGRF model is valid between the years 1900
% and 2015. See the health warning for the IGRF model here:
% http://www.ngdc.noaa.gov/IAGA/vmod/igrfhw.html
% 
% Reference:
% International Association of Geomagnetism and Aeronomy, Working Group 
% V-MOD (2010), International Geomagnetic Reference Field: the eleventh
% generation, _Geophys. J. Int._, _183_(3), 1216-1230, 
% doi:10.1111/j.1365-246X.2010.04804.x.
% 
% Inputs:
%   -TIME: Time to get the magnetic field values either in MATLAB serial
%   date number format or a string that can be converted into MATLAB serial
%   date number format using DATENUM with no format specified (see
%   documentation of DATENUM for more information).
%   -COEFS: Instead of inputting a time, you can simply specify the proper
%   coefficients for the time you want by inputting in the first argument
%   the proper coefficient vector from igrfcoefs.mat.
%   -LATITUDE: Geocentric or geodetic latitude in degrees. **SCODIN**In radian
%   -LONGITUDE: Geocentric or geodetic longitude in degrees. **SCODIN**In radian
%   -ALTITUDE: For geodetic coordiates, the height in km above the Earth's
%   surface. For geocentric coordiates, the radius in km from the center of
%   the Earth.
%   -COORD: String specifying the coordinate system to use. Either
%   'geocentric' or 'geodetic' (optional, default is geodetic). Note that
%   only geodetic coordinates have been verified.
% 
% Outputs:
%   -BX: Northward component of the magnetic field in nanoteslas (nT).
%   -BY: Eastward component of the magnetic field in nT.
%   -BZ: Downward component of the magnetic field in nT.
%   -B: [BX(:), BY(:), BZ(:)].
% 
% See also: LOADIGRFCOEFS, GETIGRFCOEFS, IGRFLINE, DATENUM, IGRF11MAGM.

% Run IGRFS if all position inputs are scalars.
if isscalar(latitude) && isscalar(longitude) && isscalar(altitude)
        [Bn, Be, Bd] = igrfs(latitude, longitude, altitude);
end

if nargout <= 1
    Bn = [Bn(:), Be(:), Bd(:)];
end
%%%%%%%%%%%%%%%%%%%%%%%%%%%%%%%%%%%%%%%%%%%%%%%%%%%%%%%%%%%%%%%%%%%%%%%%%%%
%%%%%%%%%%%%%%%%%%%        IGRF scalar function.        %%%%%%%%%%%%%%%%%%%
%%%%%%%%%%%%%%%%%%%%%%%%%%%%%%%%%%%%%%%%%%%%%%%%%%%%%%%%%%%%%%%%%%%%%%%%%%%
function [Bn, Be, Bd] = igrfs(latitude, longitude, altitude)

% Fundamental constant.
Rearth_km = 6371.2;

%%% CHECK INPUT VALIDITY %%%
% Convert time to a datenumber if it is a string.
% if ischar(time)
%     time = datenum(time);
% end

% Check that the input coordinates are scalars.
if ~isscalar(latitude) || ~isscalar(longitude) || ~isscalar(altitude)
    error('igrf1:inputNotScalar', ...
        'The input coordinates must be scalars.');
end

%%% SPHERICAL COORDINATE CONVERSION %%%
% Convert the latitude, longitude, and altitude coordinates input into
% spherical coordinates r (radius), theta (inclination angle from +z axis),
% and phi (azimuth angle from +x axis).
% We want cos(theta) and sin(theta) rather than theta itself.
costheta = cos(((pi()/2) - latitude));
sintheta = sin(((pi()/2) - latitude));

% Convert from geodetic coordinates to geocentric coordinates if necessary.
% This method was adapted from igrf11syn, which was a conversion of the
% IGRF subroutine written in FORTRAN.

r = altitude;

% Convert longitude to radians.
phi = longitude; %Conversion in Simulink

%IGRF Coefficient

gh = [-29442	-1501	4797.1	-2445.1	3012.9	-2845.6	1676.7	-641.9	1350.7	-2352.3	-115.3	1225.6	244.9	582	-538.4	907.6	813.7	283.3	120.4	-188.7	-334.9	180.9	70.4	-329.5	-232.6	360.1	47.3	192.4	197	-140.9	-119.3	-157.5	16	4.1	100.2	70	67.7	-20.8	72.7	33.2	-129.9	58.9	-28.9	-66.7	13.2	7.3	-70.9	62.6	81.6	-76.1	-54.1	-6.8	-19.5	51.8	5.7	15	24.4	9.4	3.4	-2.8	-27.4	6.8	-2.2	24.2	8.8	10.1	-16.9	-18.3	-3.2	13.3	-20.6	-14.6	13.4	16.2	11.7	5.7	-15.9	-9.1	-2	2.1	5.4	8.8	-21.6	3.1	10.8	-3.3	11.8	0.7	-6.8	-13.3	-6.9	-0.1	7.8	8.7	1	-9.1	-4	-10.5	8.4	-1.9	-6.3	3.2	0.1	-0.4	0.5	4.6	-0.5	4.4	1.8	-7.9	-0.7	-0.6	2.1	-4.2	2.4	-2.8	-1.8	-1.2	-3.6	-8.7	3.1	-1.5	-0.1	-2.3	2	2	-0.7	-0.8	-1.1	0.6	0.8	-0.7	-0.2	0.2	-2.2	1.7	-1.4	-0.2	-2.5	0.4	-2	3.5	-2.4	-1.9	-0.2	-1.1	0.4	0.4	1.2	1.9	-0.8	-2.2	0.9	0.3	0.1	0.7	0.5	-0.1	-0.3	0.3	-0.4	0.2	0.2	-0.9	-0.9	-0.1	0	0.7	0	-0.9	-0.9	0.4	0.4	0.5	1.6	-0.5	-0.5	1	-1.2	-0.2	-0.1	0.8	0.4	-0.1	-0.1	0.3	0.4	0.1	0.5	0.5	-0.3	-0.4	-0.4	-0.3	-0.8];
gh = transpose(gh);
nmax = sqrt(numel(gh) + 1) - 1;
% We need cos(m*phi) and sin(m*phi) multiple times, so precalculate into a
% vector here:
cosphi = cos((1:nmax)*phi);
sinphi = sin((1:nmax)*phi);

Pmax = (nmax+1)*(nmax+2)/2;

%%% BEGIN MAGNETIC FIELD CALCULATION %%%
% Initialize variables used in for loop below.
Br = 0; Bt = 0; Bp = 0;
 P = zeros(1, Pmax);  P(1) = 1;  P(3) = sintheta;
dP = zeros(1, Pmax); dP(1) = 0; dP(3) = costheta;

% For this initial condition, the first if will result in n = 1, m = 0.
m = 1; n = 0; coefindex = 1;

a_r = (Rearth_km/r)^2;

% Increment through all the n's and m's. gh will be a vector with g
% followed by h for incrementing through n and m except when h would be
% redundant (i.e., when m = 0).
for Pindex = 2:Pmax
    
    % Increment to the next n when m becomes larger than n.
    if n < m
        m = 0;
        n = n + 1;
        a_r = a_r*(Rearth_km/r); % We need (Rearth_km./r)^(n+2)
    end
    
    % Calculate P and dP. They are given recursively according to:
    % 
    % P(0, 0) = 1, P(1, 1) = sin(theta) <- Specified above
    % P(n, n) = sqrt(1 - 1/(2n))*sin(theta)*P(n-1, n-1)
    % P(n, m) = (2n - 1)/sqrt(n^2 - m^2)*cos(theta)*P(n-1, m) -
    %     sqrt(((n-1)^2 - m^2) / (n^2 - m^2)) * P(n-2, m)
    % 
    % dP(0, 0) = 0, dP(1, 1) = cos(theta) <- Specified above
    % dP(n, n) = sqrt(1 - 1/(2n))*(sin(theta)*dP(n-1, n-1) +
    %     cos(theta)*P(n-1, n-1))
    % dP(n, m) = (2n - 1)/sqrt(n^2 - m^2)*(cos(theta)*dP(n-1, m) -
    %     sin(theta)*P(n-1, m)) - sqrt(((n-1)^2 - m^2)/(n^2 - m^2))*
    %     dP(n-2, m)
    if m < n && Pindex ~= 3 % (Pindex=3 is n=1, m=1, initial cond. above)
        last1n = Pindex - n;
        last2n = Pindex - 2*n + 1;
        P(Pindex) = (2*n - 1)/sqrt(n^2 - m^2)*costheta*P(last1n) - ...
            sqrt(((n-1)^2 - m^2) / (n^2 - m^2)) * P(last2n);
        dP(Pindex) = (2*n - 1)/sqrt(n^2 - m^2)*(costheta*dP(last1n) - ...
            sintheta*P(last1n)) - sqrt(((n-1)^2 - m^2) / (n^2 - m^2)) * ...
            dP(last2n);
    elseif Pindex ~= 3
        lastn = Pindex - n - 1;
        P(Pindex) = sqrt(1 - 1/(2*m))*sintheta*P(lastn);
        dP(Pindex) = sqrt(1 - 1/(2*m))*(sintheta*dP(lastn) + ...
            costheta*P(lastn));
    end
    
    % Calculate the magnetic field components as a running sum. Find
    % explicit expressions for these in Global Earth Physics: a Handbook of
    % Physical Constants by Thomas J. Aherns (1995), pg. 49. Link:
    % http://books.google.com/books?id=aqjU_NHyre4C&lpg=PP1&dq=Global%20
    % earth%20physics%3A%20a%20handbook%20of%20physical%20constants&pg=PA49
    % #v=onepage&q&f=false
    % (except equation 6 is missing a required 1/sin(theta) and m; correct
    % equations on page 5 (equations 3a-3c) of:
    % http://hanspeterschaub.info/Papers/UnderGradStudents/
    % MagneticField.pdf)
    if m == 0 % Implies h = 0, so only coefficient in gh is g
        coef = a_r*gh(coefindex); %*cos(0*phi) = 1
        Br = Br + (n+1)*coef*P(Pindex);
        Bt = Bt - coef*dP(Pindex);
        % Bp is 0 for m = 0.
        coefindex = coefindex + 1; % Only need to skip over g this time.
    else
        coef = a_r*(gh(coefindex)*cosphi(m) + gh(coefindex+1)*sinphi(m));
        Br = Br + (n+1)*coef*P(Pindex);
        Bt = Bt - coef*dP(Pindex);
        if sintheta == 0 % Use different formula when dividing by 0.
            Bp = Bp - costheta*a_r*(-gh(coefindex)*sinphi(m) + ...
                gh(coefindex+1)*cosphi(m))*dP(Pindex);
        else
            Bp = Bp - 1/sintheta*a_r*m*(-gh(coefindex)*sinphi(m) + ...
                gh(coefindex+1)*cosphi(m))*P(Pindex);
        end
        coefindex = coefindex + 2; % Skip over g and h this time.
    end
    
    % Increment m.
    m = m + 1;
    
end

% Convert from spherical to (x,y,z) = (North,East,Down).
Bn = -Bt;
Be = Bp;
Bd = -Br;

== matlab function ADCS_model/Disturbances/ECEF to GEOD ==
  data: x input; latitude output; y input; z input; tol input; longitude output; altitude output
function [latitude, longitude, altitude] = ecef2geod(x, y, z, tol)

% ECEF2GEOD Convert ECEF coordinates to geodetic coordinates.
% 
% Usage: [LATITUDE, LONGITUDE, ALTITUDE] = ECEF2GEOD(X, Y, Z, TOL)
%     or [LATITUDE, LONGITUDE, ALTITUDE] = ECEF2GEOD(XYZ, TOL)
%     or LLA = ECEF2GEOD(X, Y, Z, TOL)
%     or LLA = ECEF2GEOD(XYZ, TOL)
% 
% Converts Earth-centered, Earth fixed (ECEF) coordinates X, Y, and Z to
% geodetic coordinates LATITUDE, LONGITUDE, and ALTITUDE. For a matrix
% input, the first dimension with length 3 is assumed to have the three
% separate X, Y, and Z inputs across it. The World Geodetic System 1984
% (WGS84) ellipsoid model of the Earth is assumed.
% 
% Inputs:
%   -X: x coordinates of the point in meters.
%   -Y: y coordinates of the point in meters.
%   -Z: z coordinates of the point in meters.
%   -TOL: Maximum error tolerance in the latitude in radians (optional,
%   default is 1e-12).
%   -XYZ: Matrix with at least one dimension with length 3, the first of
%   which corresponding to the dimension across which the three inputs
%   above go.
% 
% Ouputs:
%   -LATITUDE: Geodetic latitude in degrees.
%   -LONGITUDE: Geodetic longitude in degrees.
%   -ALTITUDE: Height above the Earth in meters.
%   -LLA: When just one output is requested, the three outputs above are
%   returned as a row vector for scalar inputs, an M-by-3 matrix for column
%   vector inputs, a 3-by-M matrix for row vector inputs, or the three
%   outputs concatenated either along the next largest dimension when the
%   inputs are separate arguments or the same dimension that the inputs
%   went across when a single matrix is input.
% 
% See also: ECEF2LLA, GEOD2ECEF.

% Input checking.
if nargin <= 2
    error(nargchk(1, 2, nargin));
    if nargin == 1
        tol = [];
    else
        tol = y;
    end
    sizex = size(x); first3 = find(sizex == 3, 1, 'first');
    x = reshape(permute(x, [first3, 1:(first3 - 1), ...
        (first3 + 1):ndims(x)]), 3, []);
    sizex(first3) = 1;
    y = reshape(x(2, :), sizex);
    z = reshape(x(3, :), sizex);
    x = reshape(x(1, :), sizex);
else
    error(nargchk(3, 4, nargin));
end
if nargin <= 3 || isempty(tol)
    tol = 1e-12;
end

% WGS84 parameters.
a = 6378137; f = 1/298.257223563; b = a*(1 - f); e2 = 1 - (b/a)^2;

% Longitude is easy:
longitude = atan2(y, x)*180/pi;

% Compute latitude recursively.
rd = hypot(x, y);
[latitude, Nphi] = recur(asin(z ./ hypot(x, hypot(y, z))), z, a, e2, ...
    rd, tol, 1);
sinlat = sin(latitude); coslat = cos(latitude); latitude = latitude*180/pi;

% Get altitude from latitude.
altitude = rd.*coslat + (z + e2*Nphi.*sinlat).*sinlat - Nphi;

% Shape output according to number of arguments.
if nargout <= 1
    if nargin <= 2
        latitude = cat(first3, latitude, longitude, altitude);
    else
        dims = ndims(latitude);
        if dims == 2
            if size(latitude, 2) == 1
                latitude = [latitude, longitude, altitude];
            else
                latitude = [latitude; longitude; latitude];
            end
        else
            latitude = cat(dims + 1, latitude, longitude, altitude);
        end
    end
end

function [latitude, Nphi] = recur(lat_in, z, a, e2, rd, tol, iter)
thisNphi = a ./ sqrt(1 - e2*sin(lat_in).^2);
nextlat = atan((z + thisNphi*e2.*sin(lat_in))./rd);
if all(abs(lat_in - nextlat) < tol) || iter > 100
    latitude = nextlat; Nphi = thisNphi;
else
    [latitude, Nphi] = recur(nextlat, z, a, e2, rd, tol, iter + 1);
end

== matlab function ADCS_model/Disturbances/ATMOSPHERIC DRAG/MATLAB Function ==
  data: h input; rho output
function rho = fcn(h)

%Reference altitude (km)

h_ref =linspace(250,500,7);

%Reference density (kg/m3)

rho_ref = [7.3e-11 4.1e-11 2.3e-11 1.38e-11,...
           8.33e-12 5.24e-12 3.29e-12];

%Interpolate based on altitude to find density   
       
rho = interp1(h_ref, rho_ref, h);
